simulink subsystem "acc_subsystem"  (R2025a)
settings: Solver=VariableStepAuto  StartTime=0.0  StopTime=10.0  RelTol=1e-3
settings Model: Creator=sanborkl  LastModifiedBy=sanborkl

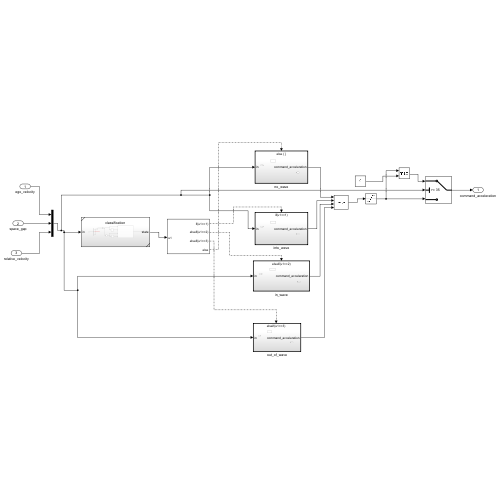
[thumbnail: Simulink's stored preview of the top-level diagram]
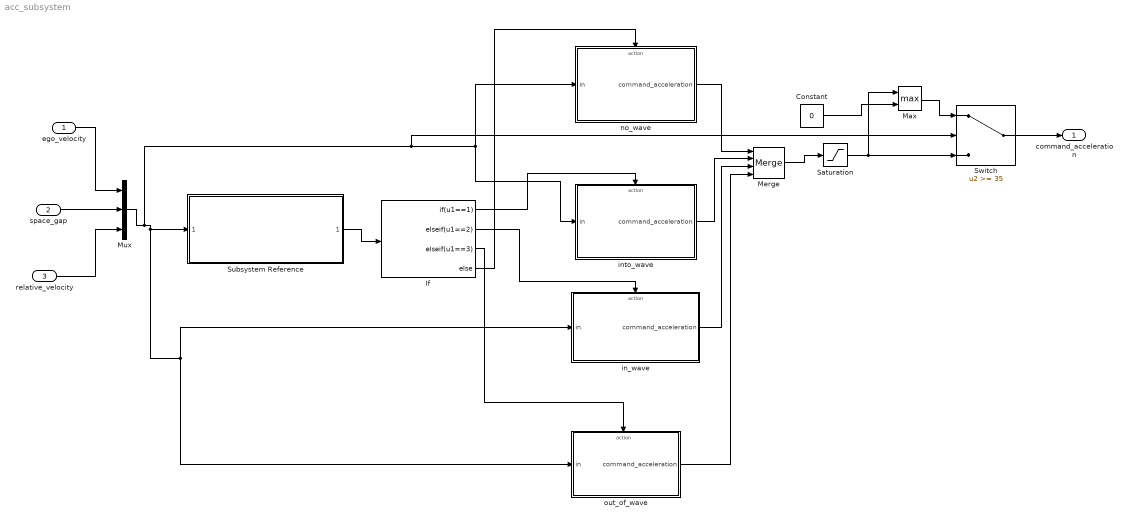
== system acc_subsystem ==
  ego_velocity : Inport
  space_gap : Inport  Port=2
  relative_velocity : Inport  Port=3
  Constant : Constant  Value=0
  If : If  IfExpression=u1==1  ElseIfExpressions=u1==2,u1==3
  Max : MinMax  Function=max  Inputs=2
  Merge : Merge  Inputs=4
  Mux : Mux  Inputs=3
  Saturation : Saturate  UpperLimit=1.5  LowerLimit=-3.0
  Subsystem Reference : Subsystem  ReferencedSubsystem=classification
  Switch : Switch  Threshold=35  SaturateOnIntegerOverflow=off  InputSameDT=off
  in_wave : Subsystem  TreatAsAtomicUnit=on
  into_wave : Subsystem  TreatAsAtomicUnit=on
  no_wave : Subsystem  TreatAsAtomicUnit=on
  out_of_wave : Subsystem  TreatAsAtomicUnit=on
  command_acceleration : Outport
  wires:
  If/2 -> in_wave/Action
  out_of_wave/1(command_acceleration) -> Merge/4
  Saturation/1 -> Max/1, Switch/3
  If/4 -> no_wave/Action
  relative_velocity/1 -> Mux/3
  If/3 -> out_of_wave/Action
  space_gap/1 -> Mux/2
  no_wave/1(command_acceleration) -> Merge/1
  If/1 -> into_wave/Action
  Subsystem Reference/1 -> If/1
  into_wave/1(command_acceleration) -> Merge/2
  Max/1 -> Switch/1
  Mux/1 -> Switch/2, into_wave/1(in), no_wave/1(in), out_of_wave/1(in), in_wave/1(in), Subsystem Reference/1
  Merge/1 -> Saturation/1
  in_wave/1(command_acceleration) -> Merge/3
  Switch/1 -> command_acceleration/1
  Constant/1 -> Max/2
  ego_velocity/1 -> Mux/1

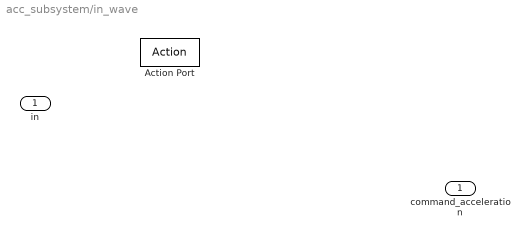
== system acc_subsystem/in_wave ==
  in : Inport
  Action Port : ActionPort  ActionPortLabel=elseif(u1==2)
  command_acceleration : Outport

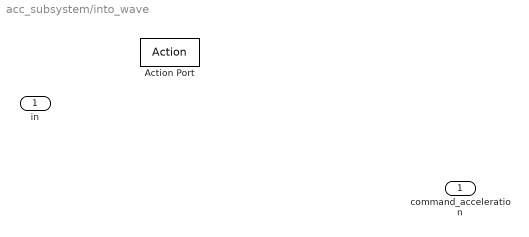
== system acc_subsystem/into_wave ==
  in : Inport
  Action Port : ActionPort  ActionPortLabel=if(u1==1)
  command_acceleration : Outport

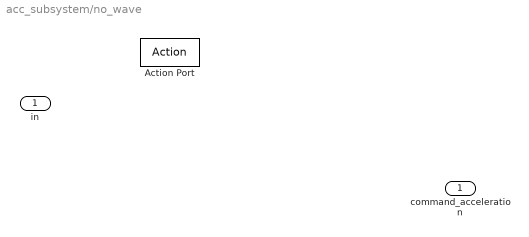
== system acc_subsystem/no_wave ==
  in : Inport
  Action Port : ActionPort  ActionPortLabel=else
  command_acceleration : Outport

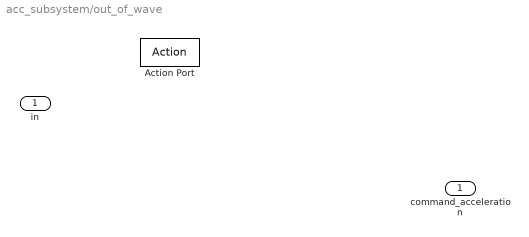
== system acc_subsystem/out_of_wave ==
  in : Inport
  Action Port : ActionPort  ActionPortLabel=elseif(u1==3)
  command_acceleration : Outport
